simulink model "zbiorniki_lin"  (R2024b)
settings: Solver=ode45  StartTime=0.0  StopTime=150  MaxStep=0.05  RelTol=1e-3
libraries: simulink x2
settings Model: Creator=lw53894  LastModifiedBy=lw53894

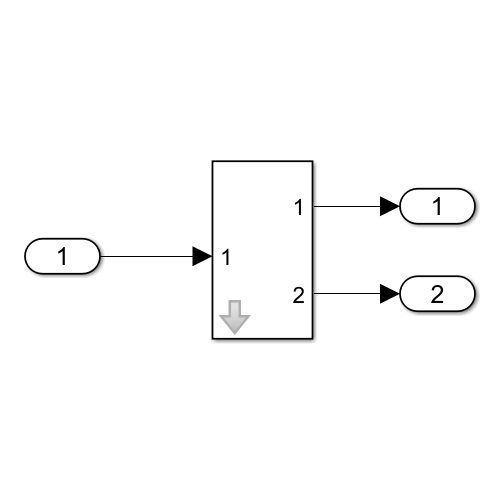
[thumbnail: Simulink's stored preview of the top-level diagram]
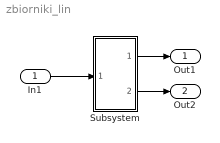
== system zbiorniki_lin ==
  In1 : Inport
  Subsystem : Subsystem  mask{h1=4, h2=2, S1=1, S2=2, Swy1=0.2, Swy2=0.2, fi1=1, fi2=1, g=9.81, Qwe=0}
  Out1 : Outport
  Out2 : Outport  Port=2
  wires:
  Subsystem/2(Out2) -> Out2/1
  Subsystem/1(Out1) -> Out1/1
  In1/1 -> Subsystem/1(In1)

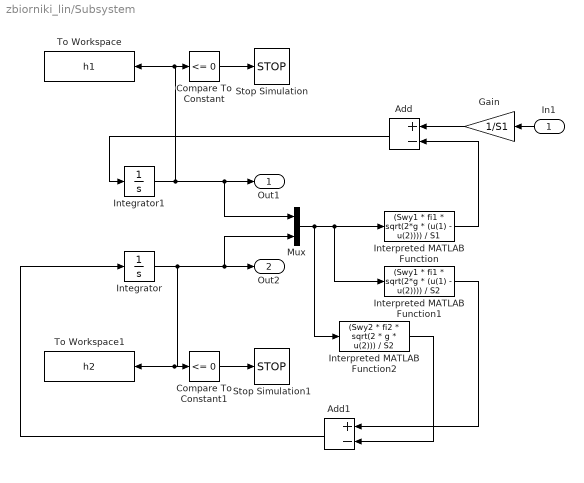
== system zbiorniki_lin/Subsystem ==
  In1 : Inport
  Add : Sum  Inputs=+-
  Add1 : Sum  Inputs=+-
  Compare To Constant : simulink/Logic and Bit Operations/Compare To Constant  relop=<=  const=0  OutDataTypeStr=boolean
  Compare To Constant1 : simulink/Logic and Bit Operations/Compare To Constant  relop=<=  const=0  OutDataTypeStr=boolean
  Gain : Gain  Gain=1/S1
  Integrator : Integrator  InitialCondition=h2
  Integrator1 : Integrator  InitialCondition=h1
  Interpreted MATLAB Function : MATLABFcn  MATLABFcn=(Swy1 * fi1 * sqrt(2*g * (u(1) - u(2)))) / S1
  Interpreted MATLAB Function1 : MATLABFcn  MATLABFcn=(Swy1 * fi1 * sqrt(2*g * (u(1) - u(2)))) / S2
  Interpreted MATLAB Function2 : MATLABFcn  MATLABFcn=(Swy2 * fi2 * sqrt(2 * g * u(2))) / S2
  Mux : Mux  Inputs=2
  Stop Simulation : Stop
  Stop Simulation1 : Stop
  To Workspace : ToWorkspace  VariableName=h1  SaveFormat=Timeseries  SampleTime=-1
  To Workspace1 : ToWorkspace  VariableName=h2  SaveFormat=Timeseries  SampleTime=-1
  Out1 : Outport
  Out2 : Outport  Port=2
  wires:
  Mux/1 -> Interpreted MATLAB Function2/1, Interpreted MATLAB Function1/1, Interpreted MATLAB Function/1
  Integrator1/1 -> To Workspace/1, Compare To Constant/1, Out1/1, Mux/1
  Integrator/1 -> To Workspace1/1, Compare To Constant1/1, Out2/1, Mux/2
  Compare To Constant/1 -> Stop Simulation/1
  Compare To Constant1/1 -> Stop Simulation1/1
  In1/1 -> Gain/1
  Add/1 -> Integrator1/1
  Interpreted MATLAB Function/1 -> Add/2
  Gain/1 -> Add/1
  Interpreted MATLAB Function1/1 -> Add1/1
  Interpreted MATLAB Function2/1 -> Add1/2
  Add1/1 -> Integrator/1
